simulink model "SOFC_model_finish"  (R2022b)
settings: Solver=VariableStepAuto  StartTime=0.0  StopTime=500  RelTol=1e-3
libraries: spsControlledVoltageSourceLib x1, spsCurrentMeasurementLib x1, spsSeriesRLCBranchLib x1, spsVoltageMeasurementLib x1, simulink x1, sps_lib x1
settings Model: Creator=86133  LastModifiedBy=86133

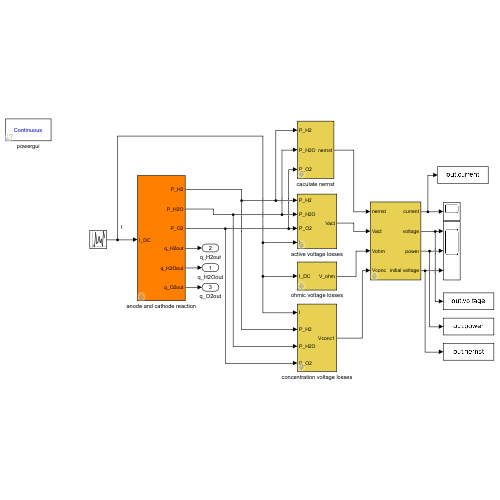
[thumbnail: Simulink's stored preview of the top-level diagram]
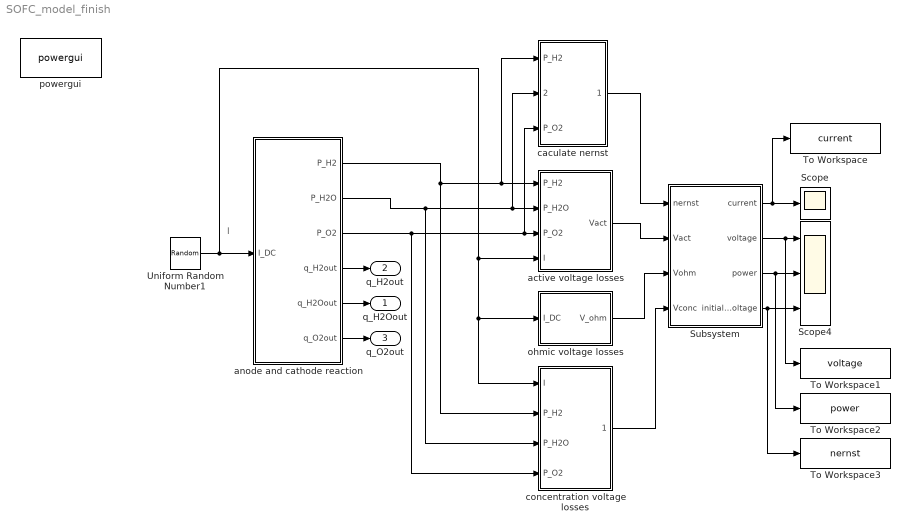
== system SOFC_model_finish ==
  note: I
  Scope : Scope
  Scope4 : Scope  NumInputPorts=3
  Subsystem : Subsystem  mask{R=8.314, F=96485, T=973, N=30, I=30, q_H2_in=0.045, K_H2=0.832, K_H2O=0.281, K_O2=2.5, rate=1.6}
      mask prompts: R "通用气体常数"; F "法拉第常数"; T "SOFC反应温度"; N "串联电池数量"; I "初始电流"; q_H2_in "氢气的输入摩尔流量"; K_H2 "氢气摩尔常数"; K_H2O "水蒸汽的摩尔常数"; K_O2 "氧气的摩尔常数"; rate "氢氧输入比例（氧：氢）"
      mask init:
      | %输入K_r
      | K_r=N/(4*F);
      | 
      | P_H2_0=1/K_H2*(q_H2_in-2*K_r*I);                   %计算氢气初始分压
      | P_O2_0=1/K_O2*(rate*q_H2_in-K_r*I);                   %计算氧气初始分压
      | P_H2O_0=1/K_O2*2*K_r*I;                   %计算水蒸气初始分压
      | 
      | nernst_init=(N*R*T)/2/F*log(P_H2_0*sqrt(P_O2_0)/P_H2O_0);
      mask DialogControl ParameterGroupVar Prompt: 参数
  To Workspace : ToWorkspace  VariableName=current  SampleTime=0.1
  To Workspace1 : ToWorkspace  VariableName=voltage  SampleTime=0.1
  To Workspace2 : ToWorkspace  VariableName=power  SampleTime=0.1
  To Workspace3 : ToWorkspace  VariableName=nernst  SampleTime=0.1
  Uniform Random Number1 : UniformRandomNumber  Minimum=15  Maximum=15.1  Seed=1  SampleTime=0.1
  active voltage losses : Subsystem  mask{Y1=5.3448*1e11, Y2=2.051*1e10, R=8.314, T=973, F=96485, I=30}
      mask prompts: Y1 "阳极交换电流密度常数γa"; Y2 "阴极交换电流密度常数γc"; R "通用气体常数"; T "SOFC运行温度"; F "法拉第常数"; I "初始电流"
      mask DialogControl DescGroupVar Prompt: %SOFC活化极化电压
      mask DialogControl DescTextVar Prompt: %计算出阳极阴极的交换电流密度，通过Butler-Volmer计算出活化极化的电压损失
      mask DialogControl ParameterGroupVar Prompt: 参数
  anode and cathode reaction : Subsystem  mask{N=30, F=96485, I=30, K_H2=0.832, K_H2O=0.281, K_O2=2.5, t_H2=26.1, t_H2O=78.3, t_O2=2.91, qH2_in=0.045, qO2_in=1.6*0.045*1, qH2_in1=0.025, qO2_in1=1.6*0.045*0.8}
      mask prompts: N "串联电池数量"; F "法拉第常数"; I "初始电流"; K_H2 "氢气摩尔常数"; K_H2O "水蒸汽的摩尔常数"; K_O2 "氧气的摩尔常数"; t_H2 "氢气的时间常数"; t_H2O "水蒸气的时间常数"; t_O2 "氧气的时间常数"; qH2_in "氢气的输入摩尔量"; qO2_in "氧气的输入摩尔量"; qH2_in1 "氢气泄露后输入摩尔量"; qO2_in1 "氧气泄露后输入摩尔量"
      mask init:
      | %输入K_r
      | K_r=N/(4*F);
      mask DialogControl DescGroupVar Prompt: %SOFC阳极阴极反应
      mask DialogControl DescTextVar Prompt: %%通过输入相关参数模拟SOFC阳极和阴极的运行情况
      mask DialogControl ParameterGroupVar Prompt: 参数
  caculate nernst : Subsystem  mask{R=8.314, F=96485, T=973, N=30, I=30, q_H2_in=0.045, K_H2=0.832, K_H2O=0.281, K_O2=2.5, rate=1.6}
      mask prompts: R "通用气体常数"; F "法拉第常数"; T "SOFC反应温度"; N "串联电池数量"; I "初始电流"; q_H2_in "氢气的输入摩尔流量"; K_H2 "氢气摩尔常数"; K_H2O "水蒸汽的摩尔常数"; K_O2 "氧气的摩尔常数"; rate "氢氧输入比例（氧：氢）"
      mask init:
      | %输入K_r
      | K_r=N/(4*F);
      | 
      | P_H2_0=1/K_H2*(q_H2_in-2*K_r*I);                   %计算氢气初始分压
      | P_O2_0=1/K_O2*(rate*q_H2_in-K_r*I);                   %计算氧气初始分压
      | P_H2O_0=1/K_O2*2*K_r*I;                   %计算水蒸气初始分压
      | 
      | nernst_init=(N*R*T)/2/F*log(P_H2_0*sqrt(P_O2_0)/P_H2O_0);
      mask DialogControl DescGroupVar Prompt: %SOFCnernst电压计算
      mask DialogControl DescTextVar Prompt: %输入通用气体常数等常数计算标准的nernst电压
      mask DialogControl ParameterGroupVar Prompt: 参数
  concentration voltage losses : Subsystem  mask{DH2_k=1e-3, DH2_H2O=1e-3, DO2_k=1e-6, DO2_N2=9*1e-5, n=0.45, m=1.5, R=8.314, T=973, la=0.005, F=96485, Pc=101325, I=30}
      mask prompts: DH2_k "氢气在阳极材料中的本征扩散系数"; DH2_H2O "氢气和水蒸气混合物的扩散系数"; DO2_k "氧气在阴极材料中的本征扩散系数"; DO2_N2 "氧气和氮气混合物的扩散系数"; n "电极的孔隙率n"; m "电极的迂曲因子m"; R "通用空气常数"; T "SOFC运行温度"; la "阳极厚度（m）"; F "法拉第常数"; Pc "阴极总压力（Pa）"; I "初始电流"
      mask DialogControl DescGroupVar Prompt: %SOFC浓差极化电压
      mask DialogControl DescTextVar Prompt: %通过计算阳极和阴极各种的极化电压
      mask DialogControl ParameterGroupVar Prompt: 参数
  ohmic voltage losses : Subsystem  mask{T=973, D=0.001}
      mask prompts: T "SOFC运行温度"; D "电解质厚度"
      mask DialogControl DescGroupVar Prompt: %SOFC欧姆极化电压
      mask DialogControl DescTextVar Prompt: %输入电解质厚度和温度参数计算得出欧姆极化电压的值
      mask DialogControl ParameterGroupVar Prompt: 参数
  powergui : sps_lib/powergui  Priority=1  SimulationMode=Continuous  SampleTime=50e-6  frequency=60  Iterations=50  frequencyindice=0  Pbase=100e6  ErrMax=1e-4  UnitsV=kV  UnitsW=MW  buscounter=0  FunctionMessages=off  echomessages=off  EnableUseOfTLC=off  CurrentSourceSwitches=off  DisableSnubberDevices=off  DisableRonSwitches=off  DisableVfSwitches=off  DisplayEquations=off  AutomaticDiscreteSolvers=off  SolverType=Tustin/Backward Euler (TBE)  Interpol=off  ExternalGateDelay=off  methode=off  Ts=100  x0status=blocks  SPID=on  SwTol=0  HookPort=off  NonlinearTolerance=1e-4  nMaxIteration=100  ContinueOnMaxIteration=off  RestoreLinks=warning  ResistiveCurrentMeasurement=off  Frange=[0:2:500]  Ylog=off  Xlog=on  ShowGrid=off  save=off  variable=ZData  structure=0  ZoomFFT=off  StartTime=0.0  cycles=1  DisplayStyle=1  fundamental=60  FreqAxis=off  MaxFrequency=1000  frequencyindicesteady=1  RmsSteady=1  display=off
  q_H2Oout : Outport
  q_H2out : Outport  Port=2
  q_O2out : Outport  Port=3
  wires:
  anode and cathode reaction/5(q_H2Oout) -> q_H2Oout/1
  anode and cathode reaction/4(q_H2out) -> q_H2out/1
  anode and cathode reaction/6(q_O2out) -> q_O2out/1
  anode and cathode reaction/1(P_H2) -> caculate nernst/1(P_H2), active voltage losses/1(P_H2), concentration voltage losses/2(P_H2)
  anode and cathode reaction/2(P_H2O) -> concentration voltage losses/3(P_H2O), caculate nernst/2(P_H2O), active voltage losses/2(P_H2O)
  anode and cathode reaction/3(P_O2) -> concentration voltage losses/4(P_O2), caculate nernst/3(P_O2), active voltage losses/3(P_O2)
  caculate nernst/1(nernst) -> Subsystem/1(nernst)
  active voltage losses/1(Vact) -> Subsystem/2(Vact)
  ohmic voltage losses/1(V_ohm) -> Subsystem/3(Vohm)
  Subsystem/2(voltage) -> To Workspace1/1, Scope4/1
  Subsystem/3(power) -> To Workspace2/1, Scope4/2
  Subsystem/4(initial voltage) -> To Workspace3/1, Scope4/3
  Subsystem/1(current) -> To Workspace/1, Scope/1
  Uniform Random Number1/1 -> ohmic voltage losses/1(I_DC), concentration voltage losses/1(I), active voltage losses/4(I), anode and cathode reaction/1(I_DC)
  concentration voltage losses/1(Vconc1) -> Subsystem/4(Vconc)

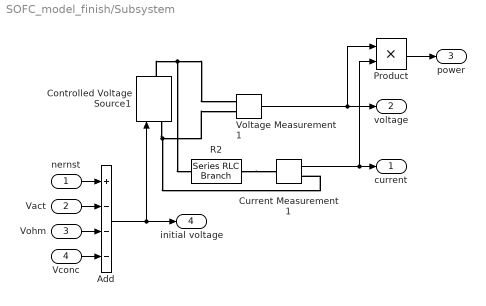
== system SOFC_model_finish/Subsystem ==
  nernst : Inport
  Vact : Inport  Port=2
  Vohm : Inport  Port=3
  Vconc : Inport  Port=4
  Add : Sum  Inputs=+---
  Controlled Voltage Source1 : spsControlledVoltageSourceLib/Controlled Voltage Source  Initialize=on  Source_Type=AC  Amplitude=nernst_init  Phase=0  Frequency=0  Measurements=None
  Current Measurement1 : spsCurrentMeasurementLib/Current Measurement  PhasorSimulation=off  OutputType=Complex  PSBequivalent=0
  Product : Product
  R2 : spsSeriesRLCBranchLib/Series RLC Branch  LConnTagsString=__new0  RConnTagsString=__new0  BranchType=R  Resistance=2  Inductance=1e-3  SetiL0=off  InitialCurrent=0  Capacitance=1e-6  Setx0=off  InitialVoltage=0  Measurements=None
  Voltage Measurement1 : spsVoltageMeasurementLib/Voltage Measurement  PhasorSimulation=off  OutputType=Complex  PSBequivalent=0
  current : Outport
  voltage : Outport  Port=2
  power : Outport  Port=3
  initial voltage : Outport  Port=4
  wires:
  Vact/1 -> Add/2
  nernst/1 -> Add/1
  Vohm/1 -> Add/3
  Add/1 -> Controlled Voltage Source1/1, initial voltage/1
  Vconc/1 -> Add/4
  Voltage Measurement1/1 -> Product/1, voltage/1
  Current Measurement1/1 -> Product/2, current/1
  Product/1 -> power/1
  connections:
  Controlled Voltage Source1/RConn1 -- R2/RConn1 -- Voltage Measurement1/LConn1
  Controlled Voltage Source1/LConn1 -- Voltage Measurement1/LConn2 -- Current Measurement1/RConn1
  R2/LConn1 -- Current Measurement1/LConn1

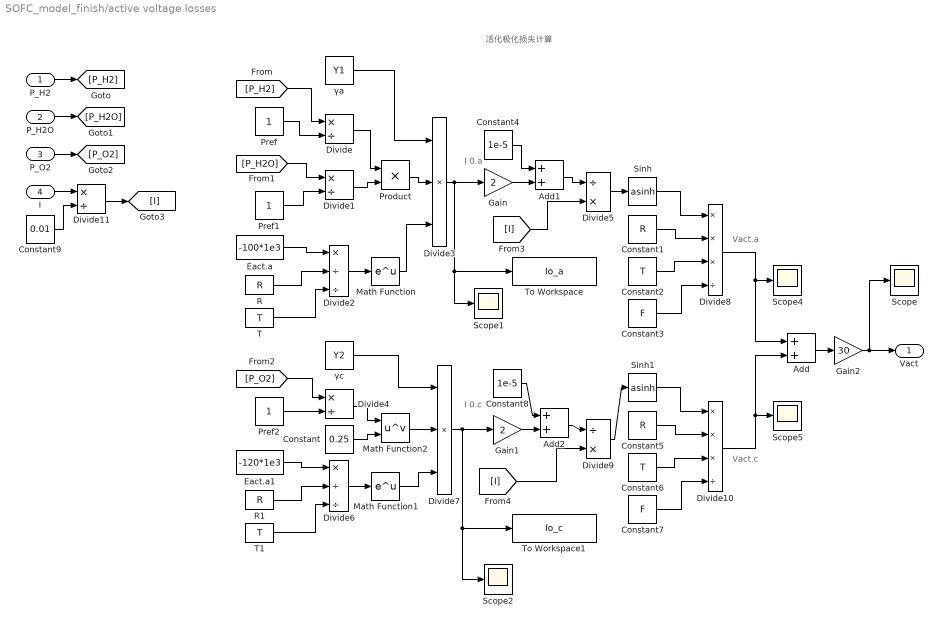
== system SOFC_model_finish/active voltage losses ==
  note: 活化极化损失计算
  note: Vact.a
  note: I 0.a
  note: I 0.c
  note: Vact.c
  P_H2 : Inport
  P_H2O : Inport  Port=2
  P_O2 : Inport  Port=3
  I : Inport  Port=4
  Add : Sum
  Add1 : Sum
  Add2 : Sum
  Constant : Constant  Value=0.25
  Constant1 : Constant  Value=R
  Constant2 : Constant  Value=T
  Constant3 : Constant  Value=F
  Constant4 : Constant  Value=1e-5
  Constant5 : Constant  Value=R
  Constant6 : Constant  Value=T
  Constant7 : Constant  Value=F
  Constant8 : Constant  Value=1e-5
  Constant9 : Constant  Value=0.01
  Divide{,1,4,11} (4 alike) : Product  Inputs=*/
  Divide10 : Product  Inputs=***/
  Divide2 : Product  Inputs=*//
  Divide3 : Product  Inputs=***
  Divide5 : Product  Inputs=/*
  Divide6 : Product  Inputs=*//
  Divide7 : Product  Inputs=***
  Divide8 : Product  Inputs=***/
  Divide9 : Product  Inputs=/*
  Eact.a : Constant  Value=-100*1e3
  Eact.a1 : Constant  Value=-120*1e3
  Gain : Gain  Gain=2
  Gain1 : Gain  Gain=2
  Gain2 : Gain  Gain=30
  Math Function : Math
  Math Function1 : Math
  Math Function2 : Math  Operator=pow
  Pref : Constant
  Pref1 : Constant
  Pref2 : Constant
  Product : Product
  R : Constant  Value=R
  R1 : Constant  Value=R
  Scope{,1..2,4..5} (5 alike) : Scope
  Sinh : Trigonometry  Operator=asinh
  Sinh1 : Trigonometry  Operator=asinh
  T : Constant  Value=T
  T1 : Constant  Value=T
  To Workspace : ToWorkspace  VariableName=Io_a  SampleTime=0.1
  To Workspace1 : ToWorkspace  VariableName=Io_c  SampleTime=0.1
  γa : Constant  Value=Y1
  γc : Constant  Value=Y2
  Vact : Outport
  wires:
  Pref/1 -> Divide/2
  Pref1/1 -> Divide1/2
  R/1 -> Divide2/2
  T/1 -> Divide2/3
  Divide2/1 -> Math Function/1
  Math Function/1 -> Divide3/3
  Divide/1 -> Product/1
  γa/1 -> Divide3/1
  P_H2/1 -> [P_H2]
  P_H2O/1 -> [P_H2O]
  [P_H2] -> Divide/1
  [P_H2O] -> Divide1/1
  [P_O2] -> Divide4/1
  T1/1 -> Divide6/3
  Divide6/1 -> Math Function1/1
  γc/1 -> Divide7/1
  R1/1 -> Divide6/2
  Pref2/1 -> Divide4/2
  Eact.a1/1 -> Divide6/1
  P_O2/1 -> [P_O2]
  Divide3/1 -> To Workspace/1, Scope1/1, Gain/1
  Divide5/1 -> Sinh/1
  Sinh/1 -> Divide8/1
  Constant1/1 -> Divide8/2
  Constant2/1 -> Divide8/3
  Constant3/1 -> Divide8/4
  Divide7/1 -> To Workspace1/1, Scope2/1, Gain1/1
  Constant7/1 -> Divide10/4
  Constant6/1 -> Divide10/3
  Constant5/1 -> Divide10/2
  Sinh1/1 -> Divide10/1
  Divide9/1 -> Sinh1/1
  Divide8/1 -> Add/1, Scope4/1
  Divide10/1 -> Scope5/1, Add/2
  Add/1 -> Gain2/1
  [I] -> Divide5/2
  [I] -> Divide9/2
  Math Function1/1 -> Divide7/3
  Math Function2/1 -> Divide7/2
  Divide4/1 -> Math Function2/1
  Constant/1 -> Math Function2/2
  Add1/1 -> Divide5/1
  Gain/1 -> Add1/2
  Constant4/1 -> Add1/1
  Add2/1 -> Divide9/1
  Gain1/1 -> Add2/2
  Constant8/1 -> Add2/1
  Divide1/1 -> Product/2
  Product/1 -> Divide3/2
  Eact.a/1 -> Divide2/1
  I/1 -> Divide11/1
  Divide11/1 -> [I]
  Constant9/1 -> Divide11/2
  Gain2/1 -> Scope/1, Vact/1

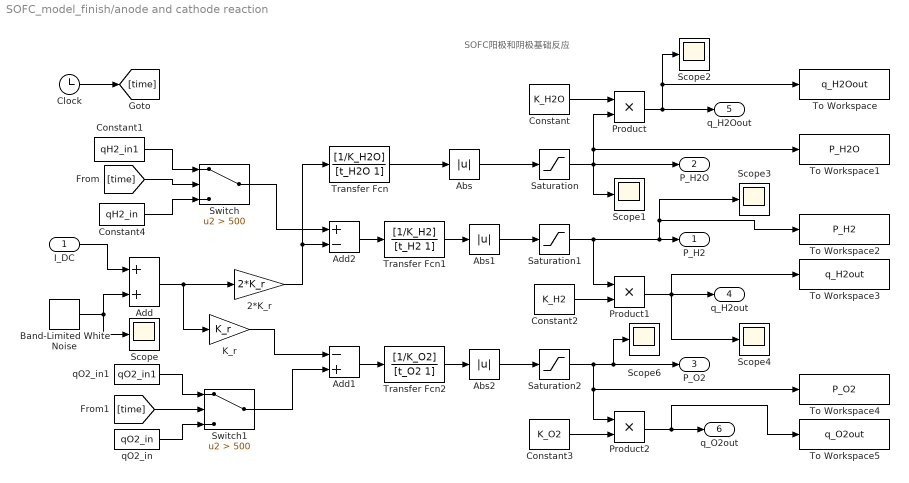
== system SOFC_model_finish/anode and cathode reaction ==
  note: SOFC阳极和阴极基础反应
  I_DC : Inport
  2*K_r : Gain  Gain=2*K_r
  Abs : Abs  SaturateOnIntegerOverflow=off
  Abs1 : Abs  SaturateOnIntegerOverflow=off
  Abs2 : Abs  SaturateOnIntegerOverflow=off
  Add : Sum
  Add1 : Sum  Inputs=-+
  Add2 : Sum  Inputs=+-
  Band-Limited White Noise : simulink/Sources/Band-Limited White Noise  Cov=[0.1*0.1]  Ts=0.1  seed=[23341]
  Clock : Clock
  Constant : Constant  Value=K_H2O
  Constant1 : Constant  Value=qH2_in1
  Constant2 : Constant  Value=K_H2
  Constant3 : Constant  Value=K_O2
  Constant4 : Constant  Value=qH2_in
  K_r : Gain  Gain=K_r
  Product : Product
  Product1 : Product
  Product2 : Product
  Saturation : Saturate  UpperLimit=1  LowerLimit=-1
  Saturation1 : Saturate  UpperLimit=1  LowerLimit=-1
  Saturation2 : Saturate  UpperLimit=1  LowerLimit=-1
  Scope{,1..4,6} (6 alike) : Scope
  Switch : Switch  Criteria=u2 > Threshold  Threshold=500  SaturateOnIntegerOverflow=off  InputSameDT=off
  Switch1 : Switch  Criteria=u2 > Threshold  Threshold=500  SaturateOnIntegerOverflow=off  InputSameDT=off
  To Workspace : ToWorkspace  VariableName=q_H2Oout  SampleTime=0.1
  To Workspace1 : ToWorkspace  VariableName=P_H2O  SampleTime=0.1
  To Workspace2 : ToWorkspace  VariableName=P_H2  SampleTime=0.1
  To Workspace3 : ToWorkspace  VariableName=q_H2out  SampleTime=0.1
  To Workspace4 : ToWorkspace  VariableName=P_O2  SampleTime=0.1
  To Workspace5 : ToWorkspace  VariableName=q_O2out  SampleTime=0.1
  Transfer Fcn : TransferFcn  Numerator=[1/K_H2O]  Denominator=[t_H2O 1]
  Transfer Fcn1 : TransferFcn  Numerator=[1/K_H2]  Denominator=[t_H2 1]
  Transfer Fcn2 : TransferFcn  Numerator=[1/K_O2]  Denominator=[t_O2 1]
  qO2_in : Constant  Value=qO2_in
  qO2_in1 : Constant  Value=qO2_in1
  P_H2 : Outport
  P_H2O : Outport  Port=2
  P_O2 : Outport  Port=3
  q_H2out : Outport  Port=4
  q_H2Oout : Outport  Port=5
  q_O2out : Outport  Port=6
  wires:
  Saturation/1 -> P_H2O/1, Scope1/1, Product/2, To Workspace1/1
  Transfer Fcn1/1 -> Abs1/1
  2*K_r/1 -> Add2/2, Transfer Fcn/1
  I_DC/1 -> Add/1
  Product2/1 -> To Workspace5/1, q_O2out/1
  Add1/1 -> Transfer Fcn2/1
  Saturation1/1 -> Product1/1, P_H2/1, To Workspace2/1, Scope3/1
  Add2/1 -> Transfer Fcn1/1
  Constant/1 -> Product/1
  Transfer Fcn2/1 -> Abs2/1
  Abs2/1 -> Saturation2/1
  Abs/1 -> Saturation/1
  Product/1 -> q_H2Oout/1, Scope2/1, To Workspace/1
  Band-Limited White Noise/1 -> Add/2, Scope/1
  Product1/1 -> To Workspace3/1, q_H2out/1, Scope4/1
  Constant3/1 -> Product2/2
  Abs1/1 -> Saturation1/1
  Transfer Fcn/1 -> Abs/1
  Constant2/1 -> Product1/2
  K_r/1 -> Add1/1
  Add/1 -> K_r/1, 2*K_r/1
  Saturation2/1 -> Scope6/1, P_O2/1, Product2/1, To Workspace4/1
  Clock/1 -> [time]
  Constant1/1 -> Switch/1
  Constant4/1 -> Switch/3
  [time] -> Switch/2
  Switch/1 -> Add2/1
  qO2_in/1 -> Switch1/3
  qO2_in1/1 -> Switch1/1
  [time] -> Switch1/2
  Switch1/1 -> Add1/2

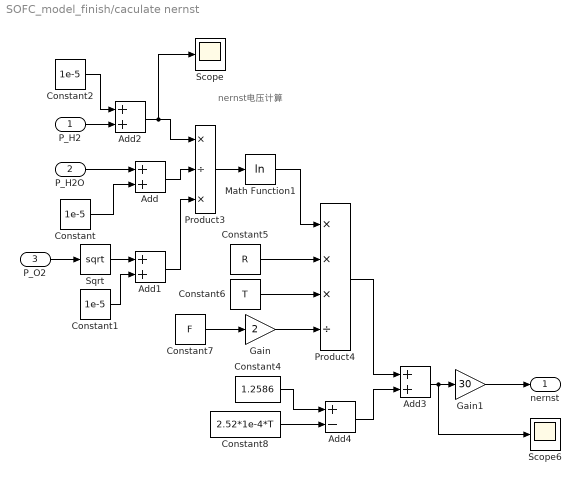
== system SOFC_model_finish/caculate nernst ==
  note: nernst电压计算
  P_H2 : Inport
  P_H2O : Inport  Port=2
  P_O2 : Inport  Port=3
  Add{,1..3} (4 alike) : Sum
  Add4 : Sum  Inputs=+-
  Constant : Constant  Value=1e-5
  Constant1 : Constant  Value=1e-5
  Constant2 : Constant  Value=1e-5
  Constant4 : Constant  Value=1.2586
  Constant5 : Constant  Value=R
  Constant6 : Constant  Value=T
  Constant7 : Constant  Value=F
  Constant8 : Constant  Value=2.52*1e-4*T
  Gain : Gain  Gain=2
  Gain1 : Gain  Gain=30
  Math Function1 : Math  Operator=log
  Product3 : Product  Inputs=*/*
  Product4 : Product  Inputs=***/
  Scope : Scope
  Scope6 : Scope
  Sqrt : Sqrt
  nernst : Outport
  wires:
  Add3/1 -> Scope6/1, Gain1/1
  Product3/1 -> Math Function1/1
  Constant7/1 -> Gain/1
  P_O2/1 -> Sqrt/1
  Math Function1/1 -> Product4/1
  Constant5/1 -> Product4/2
  Constant8/1 -> Add4/2
  P_H2O/1 -> Add/1
  Add4/1 -> Add3/2
  Constant4/1 -> Add4/1
  Product4/1 -> Add3/1
  Gain/1 -> Product4/4
  Constant6/1 -> Product4/3
  Gain1/1 -> nernst/1
  Constant/1 -> Add/2
  Add/1 -> Product3/2
  Sqrt/1 -> Add1/1
  Constant1/1 -> Add1/2
  Add1/1 -> Product3/3
  Add2/1 -> Scope/1, Product3/1
  P_H2/1 -> Add2/2
  Constant2/1 -> Add2/1

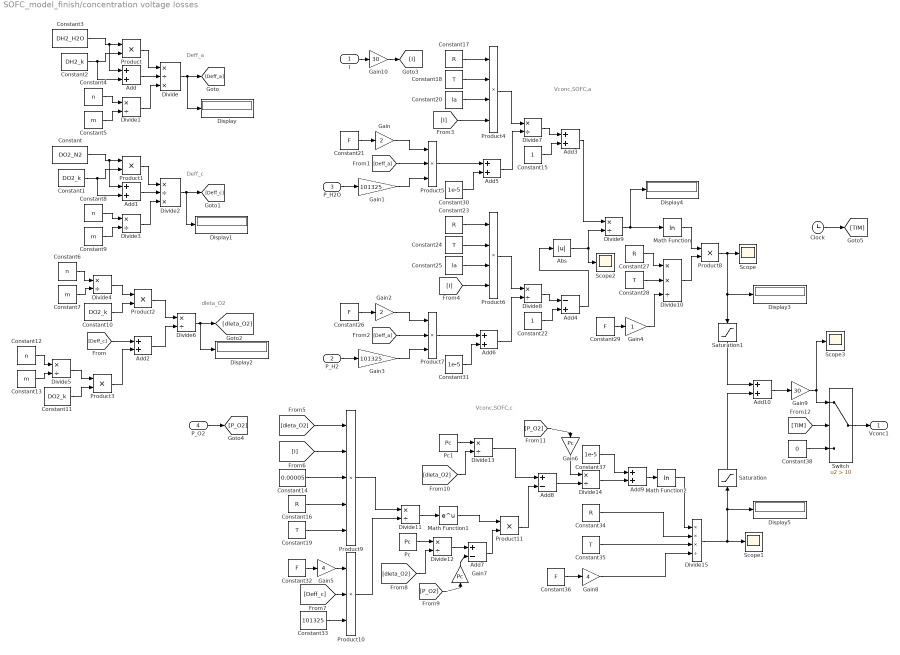
== system SOFC_model_finish/concentration voltage losses ==
  note: Vconc,SOFC,a
  note: dleta_O2
  note: Deff_c
  note: Deff_a
  note: Vconc,SOFC,c
  I : Inport
  P_H2 : Inport  Port=2
  P_H2O : Inport  Port=3
  P_O2 : Inport  Port=4
  Abs : Abs  SaturateOnIntegerOverflow=off
  Add{,1..3,5..6,9..10} (8 alike) : Sum
  Add4 : Sum  Inputs=-+
  Add7 : Sum  Inputs=+-
  Add8 : Sum  Inputs=+-
  Clock : Clock
  Constant : Constant  Value=DO2_N2
  Constant1 : Constant  Value=DO2_k
  Constant10 : Constant  Value=DO2_k
  Constant11 : Constant  Value=DO2_k
  Constant{4,6,8,12} (4 alike) : Constant  Value=n
  Constant{5,7,9,13} (4 alike) : Constant  Value=m
  Constant14 : Constant  Value=0.00005
  Constant15 : Constant
  Constant{16..17,23,27,34} (5 alike) : Constant  Value=R
  Constant{18..19,24,28,35} (5 alike) : Constant  Value=T
  Constant2 : Constant  Value=DH2_k
  Constant20 : Constant  Value=la
  Constant{21,26,29,32,36} (5 alike) : Constant  Value=F
  Constant22 : Constant
  Constant25 : Constant  Value=la
  Constant3 : Constant  Value=DH2_H2O
  Constant30 : Constant  Value=1e-5
  Constant31 : Constant  Value=1e-5
  Constant33 : Constant  Value=101325
  Constant37 : Constant  Value=1e-5
  Constant38 : Constant  Value=0
  Display{,1..5} (6 alike) : Display
  Divide : Product  Inputs=*/*
  Divide{1,3..9,11..14} (12 alike) : Product  Inputs=*/
  Divide10 : Product  Inputs=**/
  Divide15 : Product  Inputs=***/
  Divide2 : Product  Inputs=*/*
  Gain : Gain  Gain=2
  Gain1 : Gain  Gain=101325
  Gain10 : Gain  Gain=30
  Gain2 : Gain  Gain=2
  Gain3 : Gain  Gain=101325
  Gain4 : Gain
  Gain5 : Gain  Gain=4
  Gain6 : Gain  Gain=Pc
  Gain7 : Gain  Gain=Pc
  Gain8 : Gain  Gain=4
  Gain9 : Gain  Gain=30
  Math Function : Math  Operator=log
  Math Function1 : Math
  Math Function2 : Math  Operator=log
  Pc : Constant  Value=Pc
  Pc1 : Constant  Value=Pc
  Product{,1..3,8,11} (6 alike) : Product
  Product10 : Product  Inputs=3
  Product4 : Product  Inputs=4
  Product5 : Product  Inputs=3
  Product6 : Product  Inputs=4
  Product7 : Product  Inputs=3
  Product9 : Product  Inputs=5
  Saturation : Saturate  UpperLimit=1  LowerLimit=0
  Saturation1 : Saturate  UpperLimit=1  LowerLimit=0
  Scope{,1..3} (4 alike) : Scope
  Switch : Switch  Criteria=u2 > Threshold  Threshold=10  SaturateOnIntegerOverflow=off  InputSameDT=off
  Vconc1 : Outport
  wires:
  Constant3/1 -> Add/1, Product/1
  Constant2/1 -> Add/2, Product/2
  Product/1 -> Divide/1
  Add/1 -> Divide/2
  Constant4/1 -> Divide1/1
  Constant5/1 -> Divide1/2
  Divide1/1 -> Divide/3
  Divide3/1 -> Divide2/3
  Constant9/1 -> Divide3/2
  Constant8/1 -> Divide3/1
  Add1/1 -> Divide2/2
  Product1/1 -> Divide2/1
  Constant1/1 -> Product1/2, Add1/2
  Constant/1 -> Product1/1, Add1/1
  Divide/1 -> Display/1, [Deff_a]
  Divide2/1 -> Display1/1, [Deff_c]
  Constant6/1 -> Divide4/1
  Constant7/1 -> Divide4/2
  Divide4/1 -> Product2/1
  Constant10/1 -> Product2/2
  Constant11/1 -> Product3/2
  Divide5/1 -> Product3/1
  Constant13/1 -> Divide5/2
  Constant12/1 -> Divide5/1
  Product3/1 -> Add2/2
  [Deff_c] -> Add2/1
  Product2/1 -> Divide6/1
  Add2/1 -> Divide6/2
  Divide6/1 -> Display2/1, [dleta_O2]
  Constant17/1 -> Product4/1
  Constant18/1 -> Product4/2
  Constant20/1 -> Product4/3
  Constant21/1 -> Gain/1
  P_H2O/1 -> Gain1/1
  [Deff_a] -> Product5/2
  Gain/1 -> Product5/1
  Gain1/1 -> Product5/3
  Product4/1 -> Divide7/1
  Divide7/1 -> Add3/1
  Constant15/1 -> Add3/2
  Constant22/1 -> Add4/2
  Divide8/1 -> Add4/1
  Product6/1 -> Divide8/1
  Gain3/1 -> Product7/3
  Gain2/1 -> Product7/1
  [Deff_a] -> Product7/2
  P_H2/1 -> Gain3/1
  Constant26/1 -> Gain2/1
  Constant25/1 -> Product6/3
  Constant24/1 -> Product6/2
  Constant23/1 -> Product6/1
  I/1 -> Gain10/1
  [I] -> Product4/4
  [I] -> Product6/4
  Add3/1 -> Divide9/1
  Divide9/1 -> Display4/1, Math Function/1
  Constant27/1 -> Divide10/1
  Constant28/1 -> Divide10/2
  Constant29/1 -> Gain4/1
  Gain4/1 -> Divide10/3
  Math Function/1 -> Product8/1
  Divide10/1 -> Product8/2
  Product8/1 -> Scope/1, Display3/1, Saturation1/1
  Product5/1 -> Add5/1
  Add5/1 -> Divide7/2
  Constant30/1 -> Add5/2
  Add6/1 -> Divide8/2
  Product7/1 -> Add6/1
  Constant31/1 -> Add6/2
  [dleta_O2] -> Product9/1
  [I] -> Product9/2
  Constant14/1 -> Product9/3
  Constant16/1 -> Product9/4
  Constant19/1 -> Product9/5
  Constant32/1 -> Gain5/1
  Gain5/1 -> Product10/1
  [Deff_c] -> Product10/2
  Constant33/1 -> Product10/3
  Product9/1 -> Divide11/1
  Product10/1 -> Divide11/2
  Divide11/1 -> Math Function1/1
  Add4/1 -> Abs/1
  Abs/1 -> Scope2/1, Divide9/2
  Pc/1 -> Divide12/1
  [dleta_O2] -> Divide12/2
  Divide12/1 -> Add7/1
  [P_O2] -> Gain7/1
  P_O2/1 -> [P_O2]
  Math Function1/1 -> Product11/1
  Add7/1 -> Product11/2
  Product11/1 -> Add8/2
  [dleta_O2] -> Divide13/2
  Pc1/1 -> Divide13/1
  Divide13/1 -> Add8/1
  Add8/1 -> Divide14/2
  [P_O2] -> Gain6/1
  Gain6/1 -> Divide14/1
  Gain7/1 -> Add7/2
  Constant36/1 -> Gain8/1
  Math Function2/1 -> Divide15/1
  Constant34/1 -> Divide15/2
  Constant35/1 -> Divide15/3
  Gain8/1 -> Divide15/4
  Divide15/1 -> Scope1/1, Saturation/1, Display5/1
  Add9/1 -> Math Function2/1
  Divide14/1 -> Add9/2
  Constant37/1 -> Add9/1
  Add10/1 -> Gain9/1
  Gain9/1 -> Scope3/1, Switch/1
  Saturation/1 -> Add10/2
  Saturation1/1 -> Add10/1
  Clock/1 -> [TIM]
  [TIM] -> Switch/2
  Constant38/1 -> Switch/3
  Switch/1 -> Vconc1/1
  Gain10/1 -> [I]

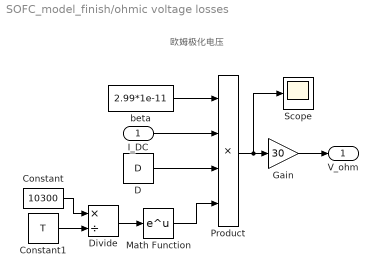
== system SOFC_model_finish/ohmic voltage losses ==
  note: 欧姆极化电压
  I_DC : Inport
  Constant : Constant  Value=10300
  Constant1 : Constant  Value=T
  D : Constant  Value=D
  Divide : Product  Inputs=*/
  Gain : Gain  Gain=30
  Math Function : Math
  Product : Product  Inputs=****
  Scope : Scope
  beta : Constant  Value=2.99*1e-11
  V_ohm : Outport
  wires:
  beta/1 -> Product/1
  I_DC/1 -> Product/2
  D/1 -> Product/3
  Constant/1 -> Divide/1
  Constant1/1 -> Divide/2
  Divide/1 -> Math Function/1
  Math Function/1 -> Product/4
  Product/1 -> Scope/1, Gain/1
  Gain/1 -> V_ohm/1
